simulink model "ExternalParadigmDemo"  (R2017a)
settings: Solver=ode45  StartTime=0.0  StopTime=inf  RelTol=1e-3  EnableMultiTasking=on
libraries: Transformation x4, Visualization x1, Amplifier x1
settings Model: ModifiedByFormat=g.tec  Creator=g.tec medical engineering  LastModifiedBy=g.tec
settings DataIOCC: LimitDataPoints=on  SaveFormat=Array
settings OptimizationCC: LifeSpan=inf
settings DebuggingCC: UnderspecifiedInitializationDetection=Classic  MergeDetectMultiDrivingBlocksExec=none  SolverPrmCheckMsg=warning  StateNameClashWarn=warning  SFUnexpectedBacktrackingDiag=warning  SFNoUnconditionalDefaultTransitionDiag=warning  SFExecutionAtInitializationDiag=none
settings HardwareCC: ProdBitPerPointer=32  ProdBitPerSizeT=32  ProdBitPerPtrDiffT=32  ProdLargestAtomicFloat=None  ProdIntDivRoundTo=Undefined  ProdEndianess=Unspecified  ProdWordSize=32  ProdHWDeviceType=32-bit Generic
settings ModelReferenceCC: PropagateSignalLabelsOutOfModel=off
settings GRTTargetCC: TargetLangStandard=C89/C90 (ANSI)  GeneratePreprocessorConditionals=Disable all
settings ConfigComp: CovMetricSettings=dw  CovHtmlReporting=on  CovSaveCumulativeToWorkspaceVar=on  CovSaveSingleToWorkspaceVar=on  CovExternalEMLEnable=off

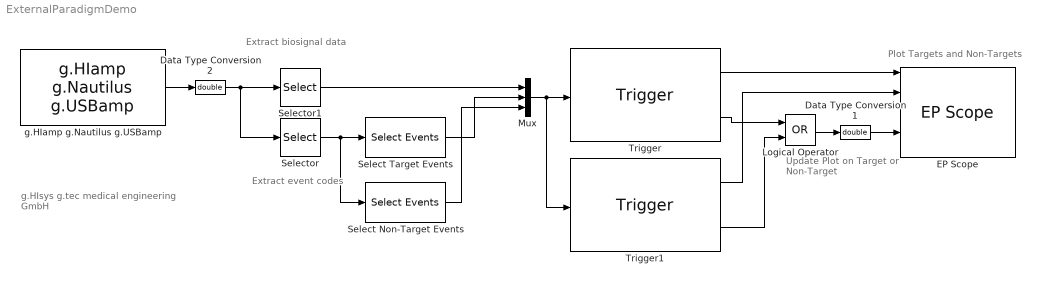
== system ExternalParadigmDemo ==
  note: Update Plot on
      | Target or Non-Target
  note: Plot Targets and Non-Targets
  note: Extract biosignal data
  note: Extract event codes
  note: g.HIsys
      | g.tec medical engineering GmbH
  Data Type Conversion1 : DataTypeConversion  OutDataTypeStr=double
  Data Type Conversion2 : DataTypeConversion  OutDataTypeStr=double
  EP Scope : Visualization/EP Scope
  Logical Operator : Logic  Operator=OR  AllPortsSameDT=off  OutDataTypeStr=boolean
  Mux : Mux  Inputs=3
  Select Non-Target Events : Transformation/Select Events  event_code=[2 4]  separate_events=off
  Select Target Events : Transformation/Select Events  event_code=[1 3 5]  separate_events=off
  Selector : Selector  InputPortWidth=2  IndexOptions=Index vector (dialog)  Indices=2  OutputSizes=1
  Selector1 : Selector  InputPortWidth=2  IndexOptions=Index vector (dialog)  Indices=1  OutputSizes=1
  Trigger : Transformation/Trigger  trigchan=2  edge_select=RISING  edge=0  treshold=1  ext_treshold=off  windowsize=0.4  pretrigger=0  sampletime=1/256  validity_select=STANDARD (global validity flag for all channels)  validity=1
  Trigger1 : Transformation/Trigger  trigchan=3  edge_select=RISING  edge=0  treshold=1  ext_treshold=off  windowsize=0.4  pretrigger=0  sampletime=1/256  validity_select=STANDARD (global validity flag for all channels)  validity=0
  g.HIamp g.Nautilus g.USBamp : Amplifier/g.HIamp g.Nautilus g.USBamp  cfgUpdated=737928.8287  numDevices=2  deviceSR=[500 250 ]  deviceChannels=[9 4 ]  numSR=[2 ]  SRIndexPerDevice=[1 0 ]
  wires:
  Select Target Events/1 -> Mux/2
  g.HIamp g.Nautilus g.USBamp/1 -> Data Type Conversion2/1
  Selector/1 -> Select Non-Target Events/1, Select Target Events/1
  Select Non-Target Events/1 -> Mux/3
  Trigger/1 -> EP Scope/1
  Trigger1/1 -> EP Scope/2
  Selector1/1 -> Mux/1
  Trigger/2 -> Logical Operator/1
  Trigger1/2 -> Logical Operator/2
  Data Type Conversion1/1 -> EP Scope/4
  Logical Operator/1 -> Data Type Conversion1/1
  Mux/1 -> Trigger1/1, Trigger/1
  Data Type Conversion2/1 -> Selector/1, Selector1/1
